simulink subsystem "PvtSubSys_DMS"  (R2020b)
settings: Solver=VariableStepAuto  StartTime=0.0  StopTime=10.0  RelTol=1e-3
undefined symbols (not defined in the file): DMS5, DS, P_DMS_tDSGoodUnbeliv2LowDistrctn, P_DMS_tDSGoodUnbeliv2LowDrowsns, P_DMS_tDSGoodUnbeliv2MidDistractn, P_DMS_tDSGoodUnbeliv2MidDrowsns, P_DMS_tDSLow2MidDistractn, P_DMS_tDSLow2MidDrowsns, P_DMS_tDSOther2Hi1Distractn, P_DMS_tDSOther2Hi1Drowsns, P_DMS_tDSOther2Hi2Distractn, P_DMS_tDSOther2Hi2Drowsns
libraries: simulink x92, TrueDurationTime x22
(part 2 of 2)

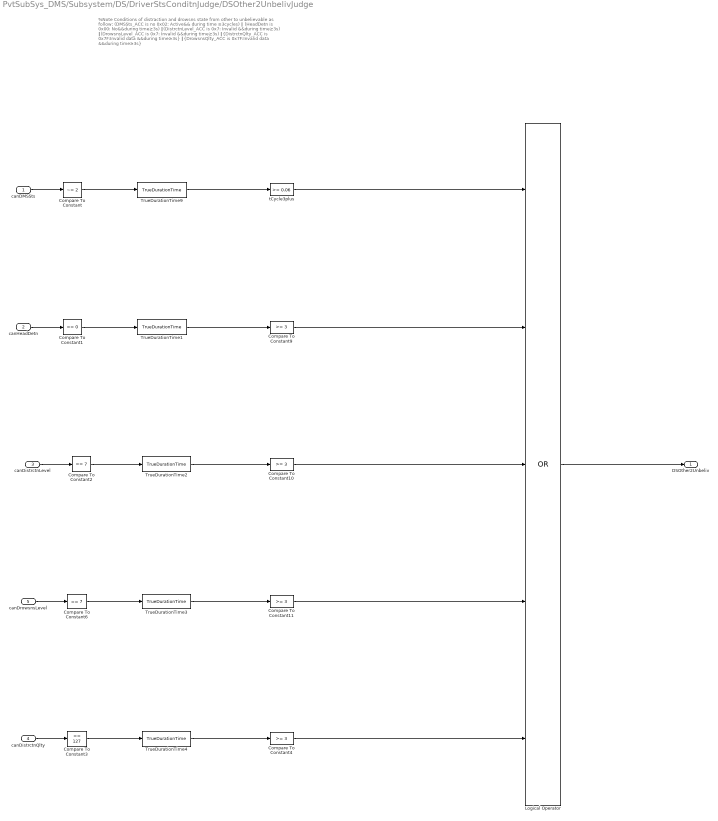
== system PvtSubSys_DMS/Subsystem/DS/DriverStsConditnJudge/DSOther2UnbelivJudge ==
  note: %Note
      | Conditions of distraction and drowsns state from other to unbelievable as follow:
      | (DMSSts_ACC is no 0x02: Active&& during time ≥3cycles)
      | ∥ (HeadDetn is 0x00: No&&during time≥3s)
      | ∥(DistrctnLevel_ACC is 0x7: Invalid &&during time≥3s)
      | ∥(DrowsnsLevel_ACC is 0x7: Invalid &&during time≥3s)
      | ∥{DistrctnQlty_ACC is 0x7F:Invalid data &&during time≥3s}
      | ∥{DrowsnsQlty_ACC is 0x7F:Invalid data &&during time≥3s}
  canDMSSts : Inport
  canHeadDetn : Inport  Port=2
  canDistrctnLevel : Inport  Port=3
  canDistrctnQlty : Inport  Port=4
  canDrowsnsLevel : Inport  Port=5
  Compare To Constant : simulink/Logic and Bit Operations/Compare To Constant  relop=~=  const=2  OutDataTypeStr=boolean
  Compare To Constant1 : simulink/Logic and Bit Operations/Compare To Constant  relop===  const=0  OutDataTypeStr=boolean
  Compare To Constant{4,9..11} (4 alike) : simulink/Logic and Bit Operations/Compare To Constant  relop=>=  const=3  OutDataTypeStr=boolean
  Compare To Constant2 : simulink/Logic and Bit Operations/Compare To Constant  relop===  const=7  OutDataTypeStr=boolean
  Compare To Constant3 : simulink/Logic and Bit Operations/Compare To Constant  relop===  const=127  OutDataTypeStr=boolean
  Compare To Constant6 : simulink/Logic and Bit Operations/Compare To Constant  relop===  const=7  OutDataTypeStr=boolean
  Logical Operator : Logic  Operator=OR  Inputs=5  AllPortsSameDT=off  OutDataTypeStr=boolean
  TrueDurationTime{1..4,9} (5 alike) : TrueDurationTime/TrueDurationTime  TCycle=0.02
  tCycle3plus : simulink/Logic and Bit Operations/Compare To Constant  relop=>=  const=0.06  OutDataTypeStr=boolean
  DSOther2Unbeliv : Outport
  wires:
  Logical Operator/1 -> DSOther2Unbeliv/1
  canDrowsnsLevel/1 -> Compare To Constant6/1
  canDistrctnQlty/1 -> Compare To Constant3/1
  canDistrctnLevel/1 -> Compare To Constant2/1
  canHeadDetn/1 -> Compare To Constant1/1
  canDMSSts/1 -> Compare To Constant/1
  Compare To Constant1/1 -> TrueDurationTime1/1
  Compare To Constant2/1 -> TrueDurationTime2/1
  Compare To Constant6/1 -> TrueDurationTime3/1
  Compare To Constant3/1 -> TrueDurationTime4/1
  Compare To Constant10/1 -> Logical Operator/3
  Compare To Constant11/1 -> Logical Operator/4
  Compare To Constant9/1 -> Logical Operator/2
  Compare To Constant4/1 -> Logical Operator/5
  tCycle3plus/1 -> Logical Operator/1
  Compare To Constant/1 -> TrueDurationTime9/1
  TrueDurationTime9/1 -> tCycle3plus/1
  TrueDurationTime1/1 -> Compare To Constant9/1
  TrueDurationTime2/1 -> Compare To Constant10/1
  TrueDurationTime3/1 -> Compare To Constant11/1
  TrueDurationTime4/1 -> Compare To Constant4/1

== system PvtSubSys_DMS/Subsystem/DS/DriverStsConditnJudge/DSUnbeliv2DDAJudge ==
  note: %Note
      | Following condition aims to prevent transition between DDA and Unbelievable constantly
      | DMSSts_ACC is 0x02: Active&&
      | HeadDetn is 0x01: Yes &&
      | DistrctnLevel_ACC is no 0x7: Invalid&&
      | DrowsnsLevel_ACC is no 0x7: Invalid&&
      | DistrctnQlty_ACC is no 0x7F:Invalid&&
      | DrowsnsQlty_ACC is no 0x7F:Invalid
  canDMSSts : Inport
  canHeadDetn : Inport  Port=2
  canDistrctnLevel : Inport  Port=3
  canDistrctnQlty : Inport  Port=4
  canDrowsnsLevel : Inport  Port=5
  Compare To Constant : simulink/Logic and Bit Operations/Compare To Constant  relop===  const=2  OutDataTypeStr=boolean
  Compare To Constant1 : simulink/Logic and Bit Operations/Compare To Constant  relop===  const=1  OutDataTypeStr=boolean
  Compare To Constant2 : simulink/Logic and Bit Operations/Compare To Constant  relop=~=  const=7  OutDataTypeStr=boolean
  Compare To Constant3 : simulink/Logic and Bit Operations/Compare To Constant  relop=~=  const=127  OutDataTypeStr=boolean
  Compare To Constant6 : simulink/Logic and Bit Operations/Compare To Constant  relop=~=  const=7  OutDataTypeStr=boolean
  Logical Operator : Logic  Inputs=5  AllPortsSameDT=off  OutDataTypeStr=boolean
  DSUnbeliv2DDAEnable : Outport
  wires:
  canDMSSts/1 -> Compare To Constant/1
  canHeadDetn/1 -> Compare To Constant1/1
  canDistrctnLevel/1 -> Compare To Constant2/1
  canDistrctnQlty/1 -> Compare To Constant3/1
  canDrowsnsLevel/1 -> Compare To Constant6/1
  Logical Operator/1 -> DSUnbeliv2DDAEnable/1
  Compare To Constant/1 -> Logical Operator/1
  Compare To Constant1/1 -> Logical Operator/2
  Compare To Constant2/1 -> Logical Operator/3
  Compare To Constant6/1 -> Logical Operator/4
  Compare To Constant3/1 -> Logical Operator/5

== stateflow chart PvtSubSys_DMS/Subsystem/DS/DriverSts_StateMachine ==
  state DriverSts [group]
    0x0:DriverUnbeliv
    0x1:DriverGood
    0x2:DriverLowDistractn
    0x3:DriverMidDistractn
    0x4:DriverHi1Distractn
    0x5:DriverHi2Distractn
    0x6:DriverLowDrowsiness
    0x7:DriverMidDrowsiness
    0x8:DriverHi1Drowsiness
    0x9:DriverHi2Drowsiness
  state DistractnSts [group]
    0x0:DMSNoDistractn
    0x1:DMSLowDistractn
    0x2:DMSMidDistractn
    0x3:DMSHi1Distractn
    0x4:DMSHi2Distractn
    0x5:DMSUnbelievDistractn
    DrowsnsSts
    0x0:DMSNoDrowsiness
    0x1:DMSLowDrowsiness
    0x2:DMSMidDrowsiness
    0x3:DMSHi1Drowsiness
    0x4:DMSHi2Drowsiness
    0x5:DMSUnbelievDrowsiness
  state Ini
    entry: DriverSts=DriverUnbeliv;
    DADistractnNoDistractn=0;
    DADrowsnsNoDrowsiness=0;
  state Unbelievable
    entry: DriverSts=DriverUnbeliv;
    DistractnSts=DMSUnbelievDistractn;
    DrowsnsSts=DMSUnbelievDrowsiness;
  state Good
    entry:DriverSts=DriverGood;
    DistractnSts=DMSNoDistractn;
    DrowsnsSts=DMSNoDrowsiness;
  state DDA
    state Distractn [parallel]
      settings: executionOrder=1
      state NoDis
        entry:DistractnSts=DMSNoDistractn;
        DADistractnNoDistractn=1;
        exit:DADistractnNoDistractn=0;
      state ExistDis
        state LowDis
          entry:DistractnSts=DMSLowDistractn;
        state MidDis
          entry:DistractnSts=DMSMidDistractn;
        state Hi1Dis
          entry:DistractnSts=DMSHi1Distractn;
        state Hi2Dis
          entry:DistractnSts=DMSHi2Distractn;
        LowDis -> (junction 143) [order 2] : [DSOther2Hi1Distractn]
        (junction 143) -> (junction 126)
        (default) -> (junction 137)
        (junction 137) -> LowDis [order 1] : [DSGoodUnbeliv2LowDistractn]
        (junction 146) -> LowDis
        (junction 147) -> (junction 146)
        (junction 137) -> (junction 142) [order 2]
        (junction 144) -> (junction 146) [order 1] : [DSMidHi1Hi22LowDistractn]
        (junction 124) -> (junction 147) [order 1] : [DSMidHi1Hi22LowDistractn]
        LowDis -> MidDis [order 1] : [DSLow2MidDistractn]
        MidDis -> LowDis [order 2] : [DSMidHi1Hi22LowDistractn]
        (junction 142) -> MidDis [order 1] : [DSGoodUnbeliv2MidDistractn]
        (junction 144) -> MidDis [order 2]
        (junction 124) -> (junction 144) [order 2]
        (junction 142) -> (junction 138) [order 2]
        Hi2Dis -> (junction 144) : [DSHi1Hi22MidDistractn||......
            | DSMidHi1Hi22LowDistractn]
        (junction 130) -> (junction 124)
        MidDis -> Hi1Dis [order 1] : [DSOther2Hi1Distractn]
        Hi1Dis -> MidDis [order 2] : [DSHi1Hi22MidDistractn]
        Hi1Dis -> Hi2Dis [order 1] : [DSOther2Hi2Distractn]
        (junction 138) -> Hi1Dis
        (junction 126) -> Hi1Dis
        Hi1Dis -> (junction 130) [order 3] : [DSHi1Hi22MidDistractn||......
            | DSMidHi1Hi22LowDistractn]
      (default) -> (junction 122)
      (junction 122) -> NoDis [order 2]
      (junction 122) -> ExistDis [order 1] : [DSGoodUnbeliv2LowDistractn||......
          | DSGoodUnbeliv2MidDistractn||......
          | DSOther2Hi1Distractn]
      NoDis -> ExistDis : [DSGoodUnbeliv2LowDistractn||......
          | DSGoodUnbeliv2MidDistractn||......
          | DSOther2Hi1Distractn]
      ExistDis -> NoDis : [DSMidHi1Hi22NoDistractn]
    state Drowsns [parallel]
      settings: executionOrder=2
      state NoDrow
        entry:DrowsnsSts=DMSNoDrowsiness;
        DADrowsnsNoDrowsiness=1;
        exit:DADrowsnsNoDrowsiness=0;
      state ExistDrow
        state LowDrow
          entry:DrowsnsSts=DMSLowDrowsiness;
        state MidDrow
          entry:DrowsnsSts=DMSMidDrowsiness;
        state Hi1Drow
          entry:DrowsnsSts=DMSHi1Drowsiness;
        state Hi2Drow
          entry:DrowsnsSts=DMSHi2Drowsiness;
        LowDrow -> (junction 58) [order 2] : [DSOther2Hi1Drowsns]
        (junction 58) -> (junction 46)
        (default) -> (junction 36)
        (junction 36) -> LowDrow [order 1] : [DSGoodUnbeliv2LowDrowsns]
        (junction 10) -> LowDrow
        (junction 74) -> (junction 10)
        (junction 36) -> (junction 42) [order 2]
        (junction 11) -> (junction 10) [order 1] : [DSMidHi1Hi22LowDrowsns]
        (junction 61) -> (junction 74) [order 1] : [DSMidHi1Hi22LowDrowsns]
        LowDrow -> MidDrow [order 1] : [DSLow2MidDrowsns]
        MidDrow -> LowDrow [order 2] : [DSMidHi1Hi22LowDrowsns]
        (junction 42) -> MidDrow [order 1] : [DSGoodUnbeliv2MidDrowsns]
        (junction 11) -> MidDrow [order 2]
        (junction 61) -> (junction 11) [order 2]
        (junction 42) -> (junction 59) [order 2]
        Hi2Drow -> (junction 11) : [DSMidHi1Hi22LowDrowsns||......
            | DSHi1Hi22MidDrowsns]
        (junction 39) -> (junction 61)
        MidDrow -> Hi1Drow [order 1] : [DSOther2Hi1Drowsns]
        Hi1Drow -> MidDrow [order 2] : [DSHi1Hi22MidDrowsns]
        Hi1Drow -> Hi2Drow [order 1] : [DSOther2Hi2Drowsns]
        (junction 59) -> Hi1Drow
        (junction 46) -> Hi1Drow
        Hi1Drow -> (junction 39) [order 3] : [DSMidHi1Hi22LowDrowsns||......
            | DSHi1Hi22MidDrowsns]
      (default) -> (junction 72)
      (junction 72) -> NoDrow [order 2]
      (junction 72) -> ExistDrow [order 1] : [DSGoodUnbeliv2LowDrowsns||......
          | DSGoodUnbeliv2MidDrowsns||......
          | DSOther2Hi1Drowsns]
      NoDrow -> ExistDrow : [DSGoodUnbeliv2LowDrowsns||......
          | DSGoodUnbeliv2MidDrowsns||......
          | DSOther2Hi1Drowsns]
      ExistDrow -> NoDrow : [DSMidHi1Hi22NoDrowsns]
    state Arbitrate [parallel]
      settings: executionOrder=3
      Arbitrate -> (junction 20)
      (junction 20) -> (junction 75) [order 1] : [DistractnSts<DrowsnsSts]
      (junction 75) -> (junction 45) [order 1] : [DrowsnsSts==DMSHi2Drowsiness]
          | {DriverSts=DriverHi2Drowsiness;}
      (junction 20) -> (junction 14) [order 2]
      (junction 75) -> (junction 54) [order 2]
      (junction 45) -> (junction 19)
      (junction 14) -> (junction 48) [order 1] : [DistractnSts==DMSHi2Distractn]
          | {DriverSts=DriverHi2Distractn;}
      (junction 54) -> (junction 19) [order 1] : [DrowsnsSts==DMSHi1Drowsiness]
          | {DriverSts=DriverHi1Drowsiness;}
      (junction 14) -> (junction 89) [order 2]
      (junction 48) -> (junction 1)
      (junction 54) -> (junction 4) [order 2]
      (junction 19) -> (junction 5)
      (junction 89) -> (junction 1) [order 1] : [DistractnSts==DMSHi1Distractn]
          | {DriverSts=DriverHi1Distractn;}
      (junction 4) -> (junction 5) [order 1] : [DrowsnsSts==DMSMidDrowsiness]
          | {DriverSts=DriverMidDrowsiness;}
      (junction 89) -> (junction 95) [order 2]
      (junction 1) -> (junction 105)
      (junction 4) -> (junction 97) [order 2] : {DriverSts=DriverLowDrowsiness;}
      (junction 5) -> (junction 102)
      (junction 95) -> (junction 105) [order 1] : [DistractnSts==DMSMidDistractn]
          | {DriverSts=DriverMidDistractn;}
      (junction 105) -> (junction 93)
      (junction 95) -> (junction 99) [order 2] : {DriverSts=DriverLowDistractn;}
      (junction 93) -> (junction 99)
      (junction 97) -> (junction 93)
      (junction 102) -> (junction 97)
      (junction 99) -> Arbitrate
  (default) -> Ini
  Ini -> Unbelievable
  Unbelievable -> Good [order 2] : [DSOther2Good]
  Good -> Unbelievable [order 1] : [DSOther2Unbeliv]
  Unbelievable -> DDA [order 1] : [(DSGoodUnbeliv2LowDistractn||......
      | DSGoodUnbeliv2MidDistractn||......
      | DSOther2Hi1Distractn||......
      | DSGoodUnbeliv2LowDrowsns||......
      | DSGoodUnbeliv2MidDrowsns||......
      | DSOther2Hi1Drowsns)&&......
      | DSUnbeliv2DDAEnable]
  DDA -> Unbelievable [order 1] : [DSOther2Unbeliv]
  DDA -> Good [order 2] : [DSOther2Good||(DADistractnNoDistractn&&DADrowsnsNoDrowsiness)]
  Good -> DDA [order 2] : [DSGoodUnbeliv2LowDistractn||......
      | DSGoodUnbeliv2MidDistractn||......
      | DSOther2Hi1Distractn||......
      | DSGoodUnbeliv2LowDrowsns||......
      | DSGoodUnbeliv2MidDrowsns||......
      | DSOther2Hi1Drowsns]
  data: DSOther2Good input; DSOther2Unbeliv input; DADistractnNoDistractn local uint8; DADrowsnsNoDrowsiness local uint8; DistractnSts output uint8 =uint8(0); DrowsnsSts output uint8 =uint8(0); DMSHi1Distractn local uint8 =uint8(3); DMSHi1Drowsiness local uint8 =uint8(3); DMSHi2Distractn local uint8 =uint8(4); DMSHi2Drowsiness local uint8 =uint8(4); DMSLowDistractn local uint8 =uint8(1); DMSLowDrowsiness local uint8 =uint8(1); DMSMidDistractn local uint8 =uint8(2); DMSMidDrowsiness local uint8 =uint8(2); DMSNoDistractn local uint8 =uint8(0); DMSNoDrowsiness local uint8 =uint8(0); DMSUnbelievDistractn local uint8 =uint8(5); DMSUnbelievDrowsiness local uint8 =uint8(5); DriverGood local uint8 =uint8(1); DriverHi1Distractn local uint8 =uint8(4); DriverHi1Drowsiness local uint8 =uint8(8); DriverHi2Distractn local uint8 =uint8(5); DriverHi2Drowsiness local uint8 =uint8(9); DriverLowDistractn local uint8 =uint8(2); DriverLowDrowsiness local uint8 =uint8(6); DriverMidDistractn local uint8 =uint8(3); DriverMidDrowsiness local uint8 =uint8(7); DriverSts output uint8; DriverUnbeliv local uint8 =uint8(0); DSGoodUnbeliv2LowDistractn input; DSMidHi1Hi22LowDistractn input; DSGoodUnbeliv2MidDistractn input; DSLow2MidDistractn input; DSHi1Hi22MidDistractn input; DSOther2Hi1Distractn input; DSOther2Hi2Distractn input; DSGoodUnbeliv2LowDrowsns input; DSMidHi1Hi22LowDrowsns input; DSGoodUnbeliv2MidDrowsns input; DSLow2MidDrowsns input; DSHi1Hi22MidDrowsns input; DSOther2Hi1Drowsns input; DSOther2Hi2Drowsns input; DSMidHi1Hi22NoDistractn input; DSMidHi1Hi22NoDrowsns input; DSUnbeliv2DDAEnable input
